simulink model "req19A"  (R2019a)
settings: Solver=FixedStepAuto  StartTime=0.0  StopTime=100  RelTol=1e-3
settings Model: Creator=e40014285  LastModifiedBy=e40014285
settings ConfigComp: CovScope=ReferencedModels  CovIncludeTopModel=off  CovHTMLOptions=-sRT=1 -sVT=0 -aTS=1 -bRG=1 -bTC=1 -hTR=0 -nFC=0 -nFD=1 -scm=1 -bcm=1 -xEv=0 -xEM=0  CovHtmlReporting=on  CovCumulativeReport=on  DVMaxProcessTime=6000  DVModelCoverageObjectives=EnhancedMCDC  DVTestSuiteOptimization=Auto  DVDetectOutOfBounds=on  DVReportPDFFormat=on  DVRebuildModelRepresentation=Always

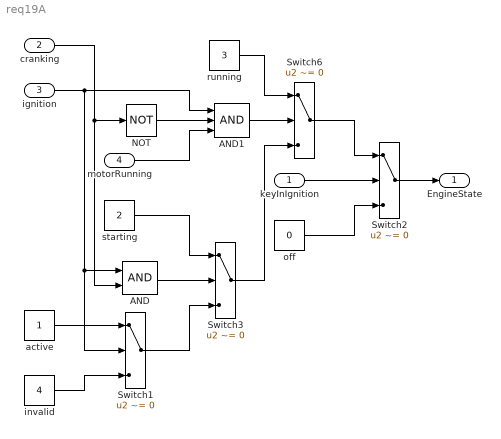
== system req19A ==
  keyInIgnition : Inport
  cranking : Inport  Port=2
  ignition : Inport  Port=3
  motorRunning : Inport  Port=4
  AND : Logic  AllPortsSameDT=off  OutDataTypeStr=boolean
  AND1 : Logic  Inputs=3  AllPortsSameDT=off  OutDataTypeStr=boolean
  NOT : Logic  Operator=NOT  AllPortsSameDT=off  OutDataTypeStr=boolean
  Switch{1..3,6} (4 alike) : Switch  Criteria=u2 ~= 0
  active : Constant
  invalid : Constant  Value=4
  off : Constant  Value=0
  running : Constant  Value=3
  starting : Constant  Value=2
  EngineState : Outport
  wires:
  motorRunning/1 -> AND1/3
  invalid/1 -> Switch1/3
  Switch3/1 -> Switch6/3
  Switch6/1 -> Switch2/1
  off/1 -> Switch2/3
  AND1/1 -> Switch6/2
  cranking/1 -> NOT/1, AND/2
  NOT/1 -> AND1/2
  Switch1/1 -> Switch3/3
  starting/1 -> Switch3/1
  AND/1 -> Switch3/2
  running/1 -> Switch6/1
  keyInIgnition/1 -> Switch2/2
  active/1 -> Switch1/1
  Switch2/1 -> EngineState/1
  ignition/1 -> AND/1, Switch1/2, AND1/1
